simulink model "test"  (R2017b)
settings: Solver=VariableStepAuto  StartTime=0.0  StopTime=100  RelTol=1e-3
undefined symbols (not defined in the file): Tp
settings Model: Creator=micha  LastModifiedBy=micha

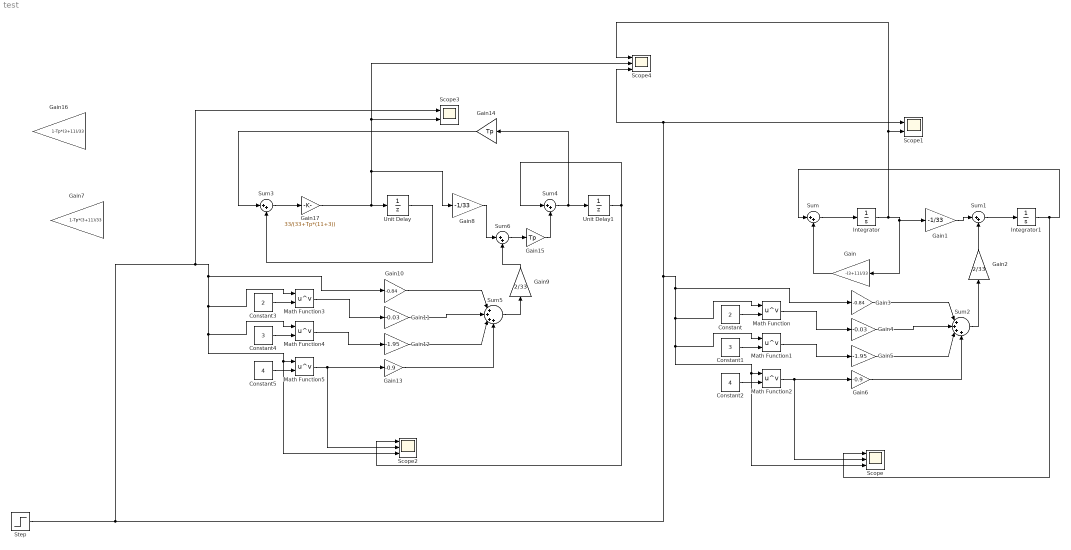
== system test ==
  Constant : Constant  Value=2
  Constant1 : Constant  Value=3
  Constant2 : Constant  Value=4
  Constant3 : Constant  Value=2
  Constant4 : Constant  Value=3
  Constant5 : Constant  Value=4
  Gain : Gain  Gain=-(3+11)/33
  Gain1 : Gain  Gain=-1/33
  Gain10 : Gain  Gain=-0.84
  Gain11 : Gain  Gain=-0.03
  Gain12 : Gain  Gain=-1.95
  Gain13 : Gain  Gain=-0.9
  Gain14 : Gain  Gain=Tp  ParamDataTypeStr=double
  Gain15 : Gain  Gain=Tp
  Gain16 : Gain  Gain=1-Tp*(3+11)/33  ParamDataTypeStr=double
  Gain17 : Gain  Gain=33/(33+Tp*(11+3))
  Gain2 : Gain  Gain=2/33
  Gain3 : Gain  Gain=-0.84
  Gain4 : Gain  Gain=-0.03
  Gain5 : Gain  Gain=-1.95
  Gain6 : Gain  Gain=-0.9
  Gain7 : Gain  Gain=1-Tp*(3+11)/33  ParamDataTypeStr=double
  Gain8 : Gain  Gain=-1/33
  Gain9 : Gain  Gain=2/33
  Integrator : Integrator
  Integrator1 : Integrator
  Math Function{,1..5} (6 alike) : Math  Operator=pow  SaturateOnIntegerOverflow=on
  Scope : Scope  NumInputPorts=3
  Scope1 : Scope  NumInputPorts=2
  Scope2 : Scope  NumInputPorts=3
  Scope3 : Scope  NumInputPorts=2
  Scope4 : Scope  NumInputPorts=3
  Step : Step  SampleTime=0
  Sum{,1,3..4,6} (5 alike) : Sum  Inputs=|++
  Sum2 : Sum  Inputs=|++++
  Sum5 : Sum  Inputs=|++++
  Unit Delay : UnitDelay  SampleTime=-1
  Unit Delay1 : UnitDelay  SampleTime=-1
  wires:
  Sum/1 -> Integrator/1
  Gain/1 -> Sum/2
  Integrator/1 -> Scope1/2, Scope4/1, Gain/1, Gain1/1
  Gain1/1 -> Sum1/1
  Sum1/1 -> Integrator1/1
  Sum2/1 -> Gain2/1
  Gain3/1 -> Sum2/1
  Gain4/1 -> Sum2/2
  Gain6/1 -> Sum2/4
  Gain5/1 -> Sum2/3
  Math Function/1 -> Gain4/1
  Math Function1/1 -> Gain5/1
  Math Function2/1 -> Scope/2, Gain6/1
  Constant/1 -> Math Function/2
  Constant1/1 -> Math Function1/2
  Gain2/1 -> Sum1/2
  Constant2/1 -> Math Function2/2
  Integrator1/1 -> Scope/1, Sum/1
  Sum4/1 -> Gain14/1, Unit Delay1/1
  Constant5/1 -> Math Function5/2
  Unit Delay/1 -> Sum3/2
  Math Function5/1 -> Scope2/2, Gain13/1
  Gain10/1 -> Sum5/1
  Constant4/1 -> Math Function4/2
  Math Function4/1 -> Gain12/1
  Math Function3/1 -> Gain11/1
  Gain12/1 -> Sum5/3
  Gain11/1 -> Sum5/2
  Unit Delay1/1 -> Sum4/1, Scope2/1
  Constant3/1 -> Math Function3/2
  Gain13/1 -> Sum5/4
  Sum5/1 -> Gain9/1
  Gain14/1 -> Sum3/1
  Gain9/1 -> Sum6/2
  Gain8/1 -> Sum6/1
  Step/1 -> Scope3/1, Gain10/1, Math Function3/1, Math Function4/1, Scope2/3, Math Function5/1, Scope1/1, Scope4/3, Gain3/1, Math Function/1, Math Function1/1, Scope/3, Math Function2/1
  Sum3/1 -> Gain17/1
  Gain17/1 -> Gain8/1, Scope3/2, Scope4/2, Unit Delay/1
  Sum6/1 -> Gain15/1
  Gain15/1 -> Sum4/2
